simulink model "Boat_Simulation_Current_demo"  (R2015a)
settings: Solver=ode3  StartTime=0.0  StopTime=50  FixedStep=dt  RelTol=1e-3
values from neighbouring files (symbols this model uses):
  airfoil_lookup = [flip(aifoil_negative_side,1);airfoil_lookup]    [boatVars.m]
  allow_disable = 1    [boatVars.m]
  ay = depth_boat*l_boat    (= 0.0096)    [boatVars.m]
  cte_disable_thresh = 100    [boatVars.m]
  d_com_aero = 0.1    [boatVars.m]
  d_motors = w_boat-0.02    (= 0.06)    [boatVars.m]
  dt = 0.1    [Analytic_Field.m]    (also in Baseline_on_Sim.m = 0.0666666666667; TrackExample.m = 0.0666666666667; TrackExample_revised.m = 0.0666666666667; boatVars.m = 0.01)
  dtor = pi/180    (= 0.0174532925199)    [boatVars.m]
  Izz_a = rho_water*((l_boat/2)^2-(w_boat/2)^2)^2*depth_boat    (= 0.0013824)    [boatVars.m]
  Izz_boat = 1    [boatVars.m]
  k_drag_rot = 0.4    [boatVars.m]
  m_boat = 0.120    (= 0.12)    [boatVars.m]
  ma_x = pi*rho_water*(w_boat/2)^2*(depth_boat)    (= 0.301592894745)    [boatVars.m]
  ma_y = pi*rho_water*(l_boat/2)^2*(depth_boat)    (= 1.20637157898)    [boatVars.m]
  rho_water = 1000    [boatVars.m]
  rot_disable_thresh = 0.0    (= 0)    [boatVars.m]
  rtod = 180/pi    (= 57.2957795131)    [boatVars.m]
  s = size(im)    [ParticleFinder.m]    (also in efficientPath.m = [50 50]; efficientPathFunc.m = [26 12]; efficientPath_newGyre.m = [s/200.*[lambda_field b_field]]; efficientPath_trials.m = [yy/2 yy/2])
  waypoints = zeros(num_waypoints,2)    [efficientPath.m]    (also in efficientPathFunc.m; efficientPath_newGyre.m)
  xd = part_pos_2(ii-1,1)    [Baseline_on_Sim.m]    (also in TrackExample.m; TrackExample_revised.m; boatVars.m = 1.5)
  xs = linspace(0,lambda_field,nx)    [boatVars.m]    (also in efficientPath_trials.m = 0:xStep:2*yy; grid_define.m = xmin:step:xmax)
  yd = part_pos_2(ii-1,2)    [Baseline_on_Sim.m]    (also in TrackExample.m; TrackExample_revised.m; boatVars.m = 0.5)
  ys = linspace(0,b_field,ny)    [boatVars.m]    (also in efficientPath_trials.m = 0:yStep:yy; grid_define.m = ymin:step:ymax)
undefined symbols (not defined in the file or in its folder): m, thrust_disable_thresh
undefined symbols (not defined in the file): alpha0_boat, b_motor, J_motor, kphi_motor, L_motor, R_motor, theta0_boat, theta_dot0_boat, v0_boat_mag, x0_boat
libraries: simulink x7, aerolib3dof2 x3, aerolibutil x2, dspmathops x2, aerolibconvert2 x2, aerolib3dofsys x1
settings Model: Creator=Jack  LastModifiedBy=Jack

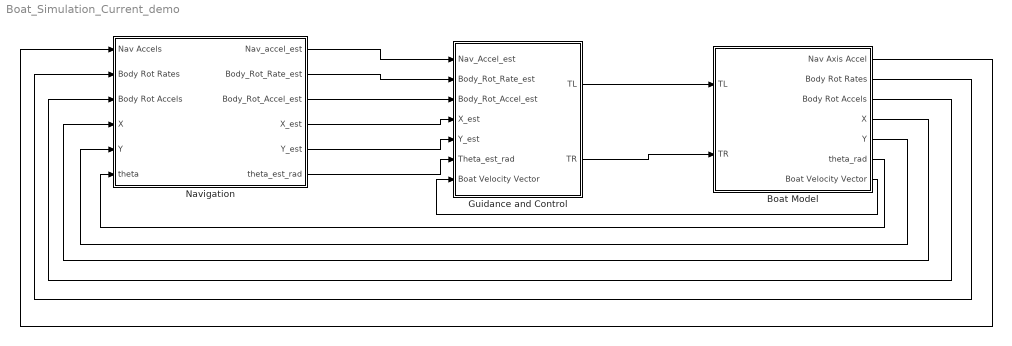
== system Boat_Simulation_Current_demo ==
  Boat Model : Subsystem
  Guidance and Control : Subsystem
  Navigation : Subsystem
  wires:
  Boat Model/1(Nav Axis Accel) -> Navigation/1(Nav Accels)
  Boat Model/2(Body Rot Rates) -> Navigation/2(Body Rot Rates)
  Boat Model/3(Body Rot Accels) -> Navigation/3(Body Rot Accels)
  Guidance and Control/1(TL) -> Boat Model/1(TL)
  Guidance and Control/2(TR) -> Boat Model/2(TR)
  Boat Model/4(X) -> Navigation/4(X)
  Boat Model/5(Y) -> Navigation/5(Y)
  Navigation/4(X_est) -> Guidance and Control/4(X_est)
  Navigation/5(Y_est) -> Guidance and Control/5(Y_est)
  Navigation/6(theta_est_rad) -> Guidance and Control/6(Theta_est_rad)
  Boat Model/6(theta_rad) -> Navigation/6(theta)
  Navigation/1(Nav_accel_est) -> Guidance and Control/1(Nav_Accel_est)
  Navigation/2(Body_Rot_Rate_est) -> Guidance and Control/2(Body_Rot_Rate_est)
  Navigation/3(Body_Rot_Accel_est) -> Guidance and Control/3(Body_Rot_Accel_est)
  Boat Model/7(Boat Velocity Vector) -> Guidance and Control/7(Boat Velocity Vector)

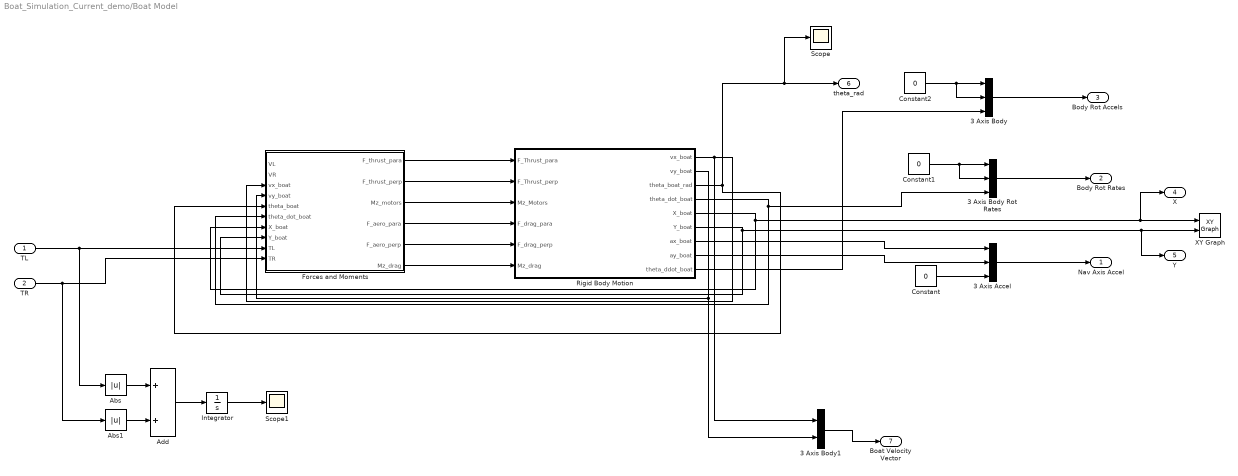
== system Boat_Simulation_Current_demo/Boat Model ==
  TL : Inport
  TR : Inport  Port=2
  3 Axis Accel : Concatenate  NumInputs=3
  3 Axis Body : Concatenate  NumInputs=3
  3 Axis Body Rot Rates : Concatenate  NumInputs=3
  3 Axis Body1 : Concatenate
  Abs : Abs
  Abs1 : Abs
  Add : Sum
  Constant : Constant  Value=0
  Constant1 : Constant  Value=0
  Constant2 : Constant  Value=0
  Forces and Moments : Subsystem
  Integrator : Integrator
  Rigid Body Motion : Subsystem
  Scope : Scope
      settings: TimeRange=10  YMin=2.71473  YMax=3.00049  SaveName=ScopeData5
  Scope1 : Scope
      settings: SaveName=ScopeData9
  XY Graph : simulink/Sinks/XY Graph  xmin=0  xmax=2  ymin=0  ymax=1  st=dt
  Nav Axis Accel : Outport
  Body Rot Rates : Outport  Port=2
  Body Rot Accels : Outport  Port=3
  X : Outport  Port=4
  Y : Outport  Port=5
  theta_rad : Outport  Port=6
  Boat Velocity Vector : Outport  Port=7
  wires:
  Forces and Moments/3(Mz_motors) -> Rigid Body Motion/3(Mz_Motors)
  Forces and Moments/2(F_thrust_perp) -> Rigid Body Motion/2(F_Thrust_perp)
  Forces and Moments/1(F_thrust_para) -> Rigid Body Motion/1(F_Thrust_para)
  Forces and Moments/4(F_aero_para) -> Rigid Body Motion/4(F_drag_para)
  Forces and Moments/5(F_aero_perp) -> Rigid Body Motion/5(F_drag_perp)
  Forces and Moments/6(Mz_drag) -> Rigid Body Motion/6(Mz_drag)
  Rigid Body Motion/1(vx_boat) -> 3 Axis Body1/1, Forces and Moments/3(vx_boat)
  Rigid Body Motion/2(vy_boat) -> 3 Axis Body1/2, Forces and Moments/4(vy_boat)
  Rigid Body Motion/3(theta_boat_rad) -> Forces and Moments/5(theta_boat), Scope/1, theta_rad/1
  Rigid Body Motion/4(theta_dot_boat) -> 3 Axis Body Rot Rates/3, Forces and Moments/6(theta_dot_boat)
  Rigid Body Motion/5(X_boat) -> Forces and Moments/7(X_boat), X/1, XY Graph/1
  Rigid Body Motion/6(Y_boat) -> Forces and Moments/8(Y_boat), Y/1, XY Graph/2
  Rigid Body Motion/7(ax_boat) -> 3 Axis Accel/1
  3 Axis Accel/1 -> Nav Axis Accel/1
  Rigid Body Motion/8(ay_boat) -> 3 Axis Accel/2
  Constant/1 -> 3 Axis Accel/3
  3 Axis Body Rot Rates/1 -> Body Rot Rates/1
  Constant1/1 -> 3 Axis Body Rot Rates/2, 3 Axis Body Rot Rates/1
  3 Axis Body/1 -> Body Rot Accels/1
  Constant2/1 -> 3 Axis Body/2, 3 Axis Body/1
  Rigid Body Motion/9(theta_ddot_boat) -> 3 Axis Body/3
  3 Axis Body1/1 -> Boat Velocity Vector/1
  TL/1 -> Abs/1, Forces and Moments/9(TL)
  TR/1 -> Abs1/1, Forces and Moments/10(TR)
  Abs/1 -> Add/1
  Abs1/1 -> Add/2
  Add/1 -> Integrator/1
  Integrator/1 -> Scope1/1

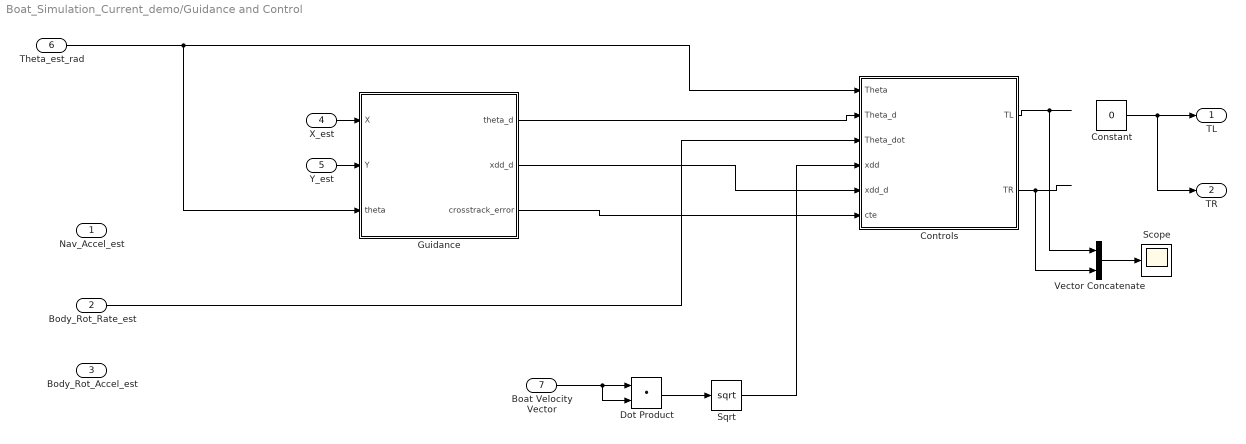
== system Boat_Simulation_Current_demo/Guidance and Control ==
  Nav_Accel_est : Inport
  Body_Rot_Rate_est : Inport  Port=2
  Body_Rot_Accel_est : Inport  Port=3
  X_est : Inport  Port=4
  Y_est : Inport  Port=5
  Theta_est_rad : Inport  Port=6
  Boat Velocity Vector : Inport  Port=7
  Constant : Constant  Value=0
  Controls : Subsystem
  Dot Product : DotProduct  InputSameDT=on  OutDataTypeStr=Inherit: Inherit via internal rule
  Guidance : Subsystem
  Scope : Scope
      settings: SaveName=ScopeData4
  Sqrt : Sqrt  SaturateOnIntegerOverflow=on
  Vector Concatenate : Concatenate
  TL : Outport
  TR : Outport  Port=2
  wires:
  Controls/1(TL) -> Vector Concatenate/1
  Controls/2(TR) -> Vector Concatenate/2
  X_est/1 -> Guidance/1(X)
  Y_est/1 -> Guidance/2(Y)
  Guidance/1(theta_d) -> Controls/2(Theta_d)
  Guidance/2(xdd_d) -> Controls/5(xdd_d)
  Theta_est_rad/1 -> Controls/1(Theta), Guidance/3(theta)
  Body_Rot_Rate_est/1 -> Controls/3(Theta_dot)
  Sqrt/1 -> Controls/4(xdd)
  Boat Velocity Vector/1 -> Dot Product/2, Dot Product/1
  Dot Product/1 -> Sqrt/1
  Vector Concatenate/1 -> Scope/1
  Guidance/3(crosstrack_error) -> Controls/6(cte)
  Constant/1 -> TR/1, TL/1

== system Boat_Simulation_Current_demo/Navigation ==
  Nav Accels : Inport
  Body Rot Rates : Inport  Port=2
  Body Rot Accels : Inport  Port=3
  X : Inport  Port=4
  Y : Inport  Port=5
  theta : Inport  Port=6
  Nav_accel_est : Outport
  Body_Rot_Rate_est : Outport  Port=2
  Body_Rot_Accel_est : Outport  Port=3
  X_est : Outport  Port=4
  Y_est : Outport  Port=5
  theta_est_rad : Outport  Port=6
  wires:
  X/1 -> X_est/1
  Y/1 -> Y_est/1
  theta/1 -> theta_est_rad/1
  Body Rot Accels/1 -> Body_Rot_Accel_est/1
  Body Rot Rates/1 -> Body_Rot_Rate_est/1
  Nav Accels/1 -> Nav_accel_est/1

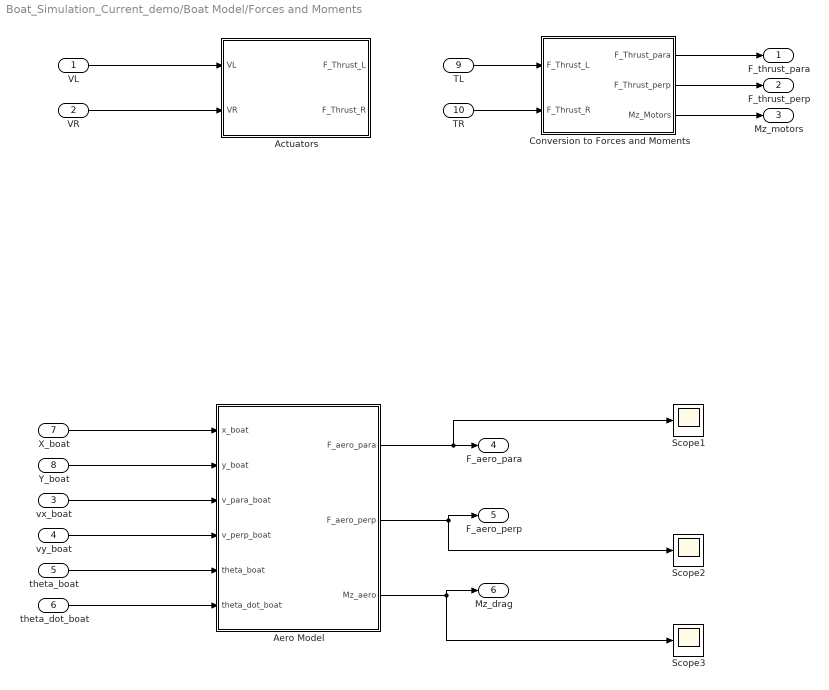
== system Boat_Simulation_Current_demo/Boat Model/Forces and Moments ==
  VL : Inport
  VR : Inport  Port=2
  vx_boat : Inport  Port=3
  vy_boat : Inport  Port=4
  theta_boat : Inport  Port=5
  theta_dot_boat : Inport  Port=6
  X_boat : Inport  Port=7
  Y_boat : Inport  Port=8
  TL : Inport  Port=9
  TR : Inport  Port=10
  Actuators : Subsystem
  Aero Model : Subsystem
  Conversion to Forces and Moments : Subsystem
  Scope1 : Scope
      settings: SaveName=ScopeData6
  Scope2 : Scope
      settings: TimeRange=10  SaveName=ScopeData8
  Scope3 : Scope
      settings: TimeRange=10  SaveName=ScopeData19
  F_thrust_para : Outport
  F_thrust_perp : Outport  Port=2
  Mz_motors : Outport  Port=3
  F_aero_para : Outport  Port=4
  F_aero_perp : Outport  Port=5
  Mz_drag : Outport  Port=6
  wires:
  VR/1 -> Actuators/2(VR)
  VL/1 -> Actuators/1(VL)
  Aero Model/3(Mz_aero) -> Scope3/1, Mz_drag/1
  Conversion to Forces and Moments/1(F_Thrust_para) -> F_thrust_para/1
  Conversion to Forces and Moments/2(F_Thrust_perp) -> F_thrust_perp/1
  Conversion to Forces and Moments/3(Mz_Motors) -> Mz_motors/1
  theta_dot_boat/1 -> Aero Model/6(theta_dot_boat)
  TL/1 -> Conversion to Forces and Moments/1(F_Thrust_L)
  TR/1 -> Conversion to Forces and Moments/2(F_Thrust_R)
  Aero Model/1(F_aero_para) -> Scope1/1, F_aero_para/1
  Aero Model/2(F_aero_perp) -> Scope2/1, F_aero_perp/1
  theta_boat/1 -> Aero Model/5(theta_boat)
  vy_boat/1 -> Aero Model/4(v_perp_boat)
  vx_boat/1 -> Aero Model/3(v_para_boat)
  Y_boat/1 -> Aero Model/2(y_boat)
  X_boat/1 -> Aero Model/1(x_boat)

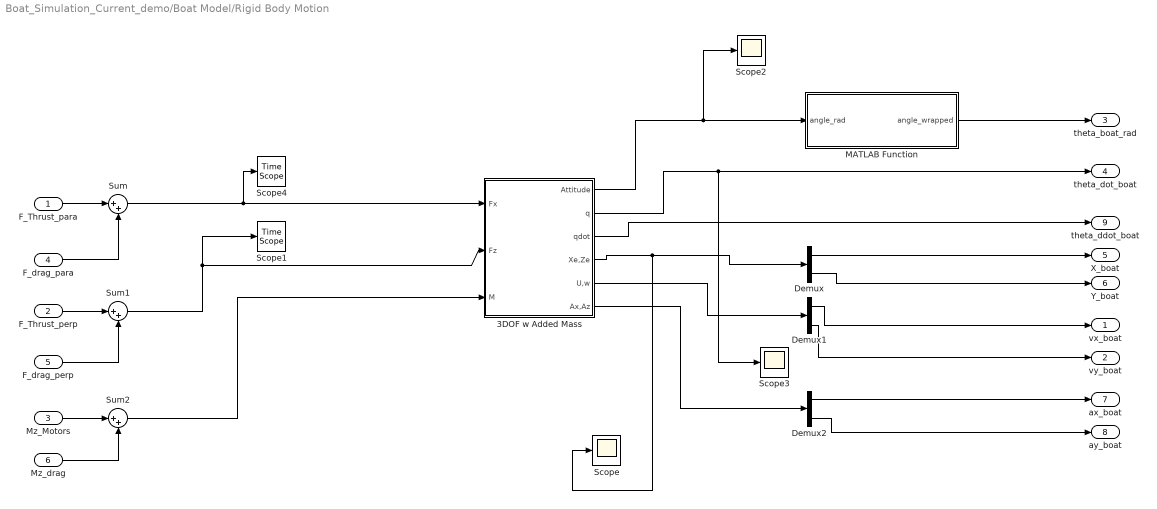
== system Boat_Simulation_Current_demo/Boat Model/Rigid Body Motion ==
  F_Thrust_para : Inport
  F_Thrust_perp : Inport  Port=2
  Mz_Motors : Inport  Port=3
  F_drag_para : Inport  Port=4
  F_drag_perp : Inport  Port=5
  Mz_drag : Inport  Port=6
  3DOF w Added Mass : Subsystem  mask(3DOF EoM){units=Metric (MKS), mtype=Fixed, v_ini=v0_boat_mag, theta_ini=theta0_boat, alpha_ini=alpha0_boat, q_ini=theta_dot0_boat, pos_ini=x0_boat, mass=m_boat, mass_e=0.5, mass_f=3.0, Iyy=Izz_boat, Iyy_e=0.5, Iyy_f=3.0, g_in=Internal, g=0, vre_flag=off}
      mask prompts: mtype "Mass type:"; v_ini "Initial velocity:"; theta_ini "Initial body attitude:"; alpha_ini "Initial incidence:"; q_ini "Initial body rotation rate:"; pos_ini "Initial position (x z):"; mass "Initial mass:"; mass_e "Empty mass:"; mass_f "Full mass:"; Iyy "Inertia:"; Iyy_e "Empty inertia:"; Iyy_f "Full inertia:"; g_in "Gravity source:"; g "Acceleration due to gravity:"; vre_flag "Include mass flow relative velocity"
      mask help: Integrate the three-degrees-of-freedom equations of motion to determine body position, velocity, attitude, and related values.
      mask init:
      | U0 = v_ini*cos(alpha_ini);
      | w0 = v_ini*sin(alpha_ini);
      | ports=aeroicon('aeroblk3dofbody','icon');
      mask Help: eval('asbhelp(''threedof_body_axes'')');
      mask TypeOptions units: Metric (MKS) | English (Velocity in ft/s) | English (Velocity in kts)
      mask TypeOptions mtype: Fixed | Simple Variable | Custom Variable
      mask Callback mtype: aeroicon('aeroblk3dofbody');
      mask TypeOptions g_in: Internal | External
      mask Callback g_in: aeroicon('aeroblk3dofbody');
      mask Display:
      | port_label(ports(1).type,ports(1).port,ports(1).txt,'texmode','on');
      | port_label(ports(2).type,ports(2).port,ports(2).txt,'texmode','on');
      | port_label(ports(3).type,ports(3).port,ports(3).txt,'texmode','on');
      | port_label(ports(4).type,ports(4).port,ports(4).txt,'texmode','on');
      | port_label(ports(5).type,ports(5).port,ports(5).txt,'texmode','on');
      | port_label(ports(6).type,ports(6).port,ports(6).txt,'texmode','on');
      | port_label(ports(7).type,ports(7).port,ports(7).txt,'texmode','on');
      | port_label(ports(8).type,ports(8).port,ports(8).txt,'texmode','on');
      | port_label(ports(9).type,ports(9).port,ports(9).txt,'texmode','on');
      | port_label(ports(10).type,ports(10).port,ports(10).txt,'texmode','on');
      | port_label(ports(11).type,ports(11).port,ports(11).txt,'texmode','on');
      | port_label(ports(12).type,ports(12).port,ports(12).txt,'texmode','on');
      | port_label(ports(13).type,ports(13).port,ports(13).txt,'texmode','on');
      | port_label(ports(14).type,ports(14).port,ports(14).txt,'texmode','on');
      | port_label(ports(15).type,ports(15).port,ports(15).txt,'texmode','on');
      | port_label(ports(16).type,ports(16).port,ports(16).txt,'texmode','on');
      | [x y xp yp highstr lowstr maxy miny]=aeroimage('threedofbody',gcbh);
      | plot(x,y);
      | patch(xp, yp);
      | text(0.5,maxy+0.08,highstr{:},'horizontalAlignment','center')
      | text(0.5,miny-0.05,lowstr{:},'horizontalAlignment','center')
  Demux : Demux  Outputs=2
  Demux1 : Demux  Outputs=2
  Demux2 : Demux  Outputs=2
  MATLAB Function : MATLAB Function  TreatAsAtomicUnit=on
  Scope : Scope
      settings: YMin=0  YMax=2
  Scope1 : TimeScope
  Scope2 : Scope
      settings: SaveName=ScopeData31
  Scope3 : Scope
      settings: SaveName=ScopeData32
  Scope4 : TimeScope
  Sum : Sum  Inputs=|++
  Sum1 : Sum  Inputs=|++
  Sum2 : Sum  Inputs=|++
  vx_boat : Outport
  vy_boat : Outport  Port=2
  theta_boat_rad : Outport  Port=3
  theta_dot_boat : Outport  Port=4
  X_boat : Outport  Port=5
  Y_boat : Outport  Port=6
  ax_boat : Outport  Port=7
  ay_boat : Outport  Port=8
  theta_ddot_boat : Outport  Port=9
  wires:
  F_drag_para/1 -> Sum/2
  Mz_Motors/1 -> Sum2/1
  Mz_drag/1 -> Sum2/2
  Demux/1 -> X_boat/1
  Demux/2 -> Y_boat/1
  Demux1/1 -> vx_boat/1
  Demux1/2 -> vy_boat/1
  Demux2/1 -> ax_boat/1
  Demux2/2 -> ay_boat/1
  MATLAB Function/1(angle_wrapped) -> theta_boat_rad/1
  3DOF w Added Mass/2("q ") -> Scope3/1, theta_dot_boat/1
  3DOF w Added Mass/3(qdot) -> theta_ddot_boat/1
  3DOF w Added Mass/1(Attitude) -> Scope2/1, MATLAB Function/1(angle_rad)
  3DOF w Added Mass/4(Xe,Ze) -> Scope/1, Demux/1
  3DOF w Added Mass/5("U,w  ") -> Demux1/1
  3DOF w Added Mass/6(Ax,Az) -> Demux2/1
  F_drag_perp/1 -> Sum1/2
  F_Thrust_para/1 -> Sum/1
  F_Thrust_perp/1 -> Sum1/1
  Sum1/1 -> Scope1/1, 3DOF w Added Mass/2(Fz)
  Sum/1 -> 3DOF w Added Mass/1(Fx), Scope4/1
  Sum2/1 -> 3DOF w Added Mass/3(M)

== system Boat_Simulation_Current_demo/Guidance and Control/Controls ==
  Theta : Inport
  Theta_d : Inport  Port=2
  Theta_dot : Inport  Port=3
  xdd : Inport  Port=4
  xdd_d : Inport  Port=5
  cte : Inport  Port=6
  Axial Control Loops : Subsystem
  Demux : Demux  Outputs=3
  Prop Allocation : Subsystem
  Rotation Control Loops : Subsystem
  TL : Outport
  TR : Outport  Port=2
  wires:
  Theta/1 -> Rotation Control Loops/1(Theta)
  Theta_d/1 -> Rotation Control Loops/2(Theta_d)
  Rotation Control Loops/1(Theta_err) -> Prop Allocation/1(theta_err)
  Prop Allocation/1(TL) -> TL/1
  Prop Allocation/2(TR) -> TR/1
  Axial Control Loops/1(xdd_err) -> Prop Allocation/2(xdd_err)
  xdd/1 -> Axial Control Loops/1(xdd)
  xdd_d/1 -> Axial Control Loops/2(xdd_d)
  Theta_dot/1 -> Demux/1
  Demux/3 -> Rotation Control Loops/3(Theta_dot_est)
  cte/1 -> Prop Allocation/3(cte)

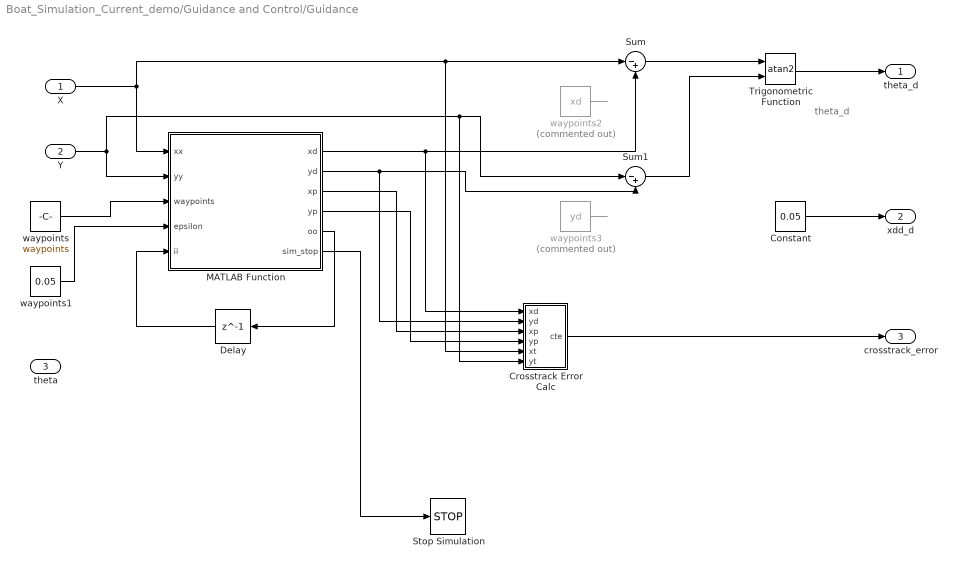
== system Boat_Simulation_Current_demo/Guidance and Control/Guidance ==
  note: theta_d
  X : Inport
  Y : Inport  Port=2
  theta : Inport  Port=3
  Constant : Constant  Value=0.05
  "Crosstrack Error Calc " : Subsystem
  Delay : Delay  DelayLength=1  InitialCondition=2
  MATLAB Function : MATLAB Function  TreatAsAtomicUnit=on
  Stop Simulation : Stop
  Sum : Sum  Inputs=|-+
  Sum1 : Sum  Inputs=|-+
  Trigonometric Function : Trigonometry  Operator=atan2
  waypoints : Constant  Value=waypoints
  waypoints1 : Constant  Value=0.05
  waypoints2 : Constant  Commented=on  Value=xd
  waypoints3 : Constant  Commented=on  Value=yd
  theta_d : Outport
  xdd_d : Outport  Port=2
  crosstrack_error : Outport  Port=3
  wires:
  X/1 -> MATLAB Function/1(xx), "Crosstrack Error Calc "/5(xt), Sum/1
  MATLAB Function/1(xd) -> Sum/2, "Crosstrack Error Calc "/1(xd)
  Sum/1 -> Trigonometric Function/1
  Sum1/1 -> Trigonometric Function/2
  Trigonometric Function/1 -> theta_d/1
  Constant/1 -> xdd_d/1
  waypoints/1 -> MATLAB Function/3(waypoints)
  waypoints1/1 -> MATLAB Function/4(epsilon)
  MATLAB Function/5(oo) -> Delay/1
  Delay/1 -> MATLAB Function/5(ii)
  waypoints2/1 -> ?
  waypoints3/1 -> ?
  MATLAB Function/6(sim_stop) -> Stop Simulation/1
  MATLAB Function/2(yd) -> Sum1/2, "Crosstrack Error Calc "/2(yd)
  MATLAB Function/3(xp) -> "Crosstrack Error Calc "/3(xp)
  MATLAB Function/4(yp) -> "Crosstrack Error Calc "/4(yp)
  "Crosstrack Error Calc "/1(cte) -> crosstrack_error/1
  Y/1 -> MATLAB Function/2(yy), "Crosstrack Error Calc "/6(yt), Sum1/1

== system Boat_Simulation_Current_demo/Boat Model/Forces and Moments/Actuators ==
  note: Left Motor
  note: Right Motor
  VL : Inport
  VR : Inport  Port=2
  DC motor : Subsystem  mask(DC Motor){L=L_motor, Kphi=kphi_motor, J=J_motor, b=b_motor, R=R_motor}
      mask help:
      | Takes the DC voltage as input, and outputs angular velocity (w) and current (i)
      | L => windings inductance		Kphi => emf constant
      | J => loads moment of inertial		b => viscous friction
      | R => windings resistance
      mask Display:
      | port_label('input', 1, 'V')
      | port_label('output', 2, 'i')
      | port_label('output', 1, 'w')
      | disp('DC Motor')
  DC motor1 : Subsystem  mask(DC Motor){L=L_motor, Kphi=kphi_motor, J=J_motor, b=b_motor, R=R_motor}
      mask help:
      | Takes the DC voltage as input, and outputs angular velocity (w) and current (i)
      | L => windings inductance		Kphi => emf constant
      | J => loads moment of inertial		b => viscous friction
      | R => windings resistance
      mask Display:
      | port_label('input', 1, 'V')
      | port_label('output', 2, 'i')
      | port_label('output', 1, 'w')
      | disp('DC Motor')
  Prop Angular Velocity to Thrust : Lookup_n-D  NumberOfTableDimensions=1  BreakpointsForDimension1=[-5:5]  Table=tanh([-5:5])  InternalRulePriority=Speed  RndMeth=Simplest  InputSameDT=on
  Prop Angular Velocity to Thrust1 : Lookup_n-D  NumberOfTableDimensions=1  BreakpointsForDimension1=[-5:5]  Table=tanh([-5:5])  InternalRulePriority=Speed  RndMeth=Simplest  InputSameDT=on
  F_Thrust_L : Outport
  F_Thrust_R : Outport  Port=2
  wires:
  DC motor/1(w) -> Prop Angular Velocity to Thrust/1
  DC motor1/1(w) -> Prop Angular Velocity to Thrust1/1
  VL/1 -> DC motor/1(V)
  VR/1 -> DC motor1/1(V)
  Prop Angular Velocity to Thrust/1 -> F_Thrust_L/1
  Prop Angular Velocity to Thrust1/1 -> F_Thrust_R/1

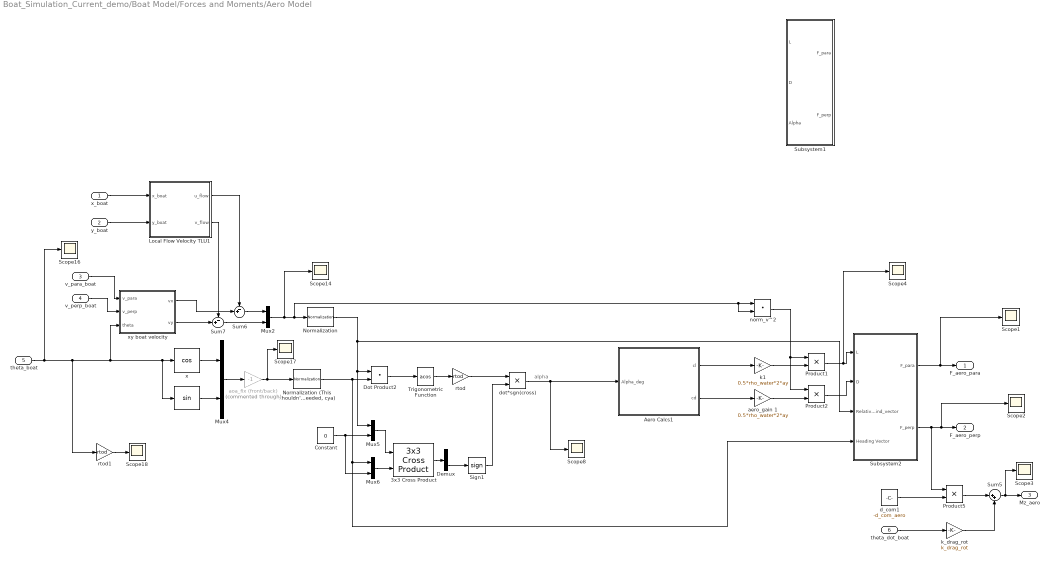
== system Boat_Simulation_Current_demo/Boat Model/Forces and Moments/Aero Model ==
  note: alpha
  x_boat : Inport
  y_boat : Inport  Port=2
  v_para_boat : Inport  Port=3
  v_perp_boat : Inport  Port=4
  theta_boat : Inport  Port=5
  theta_dot_boat : Inport  Port=6
  " " : Trigonometry
  3x3 Cross Product : aerolibutil/3x3 Cross Product
  Aero Calcs1 : Subsystem
  Constant : Constant  Value=0
  Demux : Demux  Outputs=3
  Dot Product2 : DotProduct  InputSameDT=on  OutDataTypeStr=Inherit: Inherit via internal rule
  Local Flow Velocity TLU1 : Subsystem
  Mux{2,4..6} (4 alike) : Mux  Inputs=2
  Normalization : dspmathops/Normalization  NormType=2-norm  Bias=1e-10  NormOver=Each column  ColComp=off  Dimension=1  outputDataTypeStr=Inherit: Same as product output  outputLastDataTypeStr=Inherit: Same as product output  outputMin=[]  outputMax=[]  accumDataTypeStr=Inherit: Same as product output  accumLastDataTypeStr=Inherit: Same as product output  roundingMode=Floor  overflowMode=off
  "Normalization (This shouldn't be needed, cya)" : dspmathops/Normalization  NormType=2-norm  Bias=1e-10  NormOver=Each column  ColComp=off  Dimension=1  outputDataTypeStr=Inherit: Same as product output  outputLastDataTypeStr=Inherit: Same as product output  outputMin=[]  outputMax=[]  accumDataTypeStr=Inherit: Same as product output  accumLastDataTypeStr=Inherit: Same as product output  roundingMode=Floor  overflowMode=off
  Product1 : Product
  Product2 : Product
  Product5 : Product
  Scope{1..4,8,14,16..18} (9 alike) : Scope
      Scope1 settings: YMin=-0.000475  YMax=-0.000225  SaveName=ScopeData7
      Scope14 settings: ShowLegends=on  SaveName=ScopeData24
      Scope16 settings: SaveName=ScopeData28
      Scope17 settings: ShowLegends=on  SaveName=ScopeData29
      Scope18 settings: YMin=45  YMax=45  SaveName=ScopeData30
      Scope2 settings: YMin=-1  YMax=1  SaveName=ScopeData10
      Scope3 settings: YMin=-1  YMax=1  SaveName=ScopeData11
      Scope4 settings: ShowLegends=on  YMin=-0.005  YMax=0.075  SaveName=ScopeData16
      Scope8 settings: YMin=-141.75  YMax=-128.25  SaveName=ScopeData26
  Sign1 : Signum
  Subsystem1 : Subsystem
  Subsystem2 : Subsystem
  Sum5 : Sum  Inputs=|++
  Sum6 : Sum  Inputs=-+|
  Sum7 : Sum  Inputs=-+|
  Trigonometric Function : Trigonometry  Operator=acos
  aero_gain 1 : Gain  Gain=0.5*rho_water*2*ay
  aoa_fix (front/back) : Gain  Commented=through  Gain=-1
  d_com1 : Constant  Value=-d_com_aero
  dot*sgn(cross) : Product
  k1 : Gain  Gain=0.5*rho_water*2*ay
  k_drag_rot : Gain  Gain=k_drag_rot
  norm_v^2 : DotProduct  InputSameDT=on  OutDataTypeStr=Inherit: Inherit via internal rule
  rtod : Gain  Gain=rtod
  rtod1 : Gain  Gain=rtod
  x : Trigonometry  Operator=cos
  "xy boat velocity " : Subsystem
  F_aero_para : Outport
  F_aero_perp : Outport  Port=2
  Mz_aero : Outport  Port=3
  wires:
  x_boat/1 -> Local Flow Velocity TLU1/1(x_boat)
  y_boat/1 -> Local Flow Velocity TLU1/2(y_boat)
  Local Flow Velocity TLU1/1(u_flow) -> Sum6/1
  Local Flow Velocity TLU1/2(v_flow) -> Sum7/1
  theta_dot_boat/1 -> k_drag_rot/1
  k_drag_rot/1 -> Sum5/2
  Subsystem2/2(F_perp) -> Product5/1, Scope2/1, F_aero_perp/1
  d_com1/1 -> Product5/2
  Product5/1 -> Sum5/1
  Sum5/1 -> Scope3/1, Mz_aero/1
  theta_boat/1 -> Scope16/1, rtod1/1, "xy boat velocity "/3("theta "), " "/1, x/1
  x/1 -> Mux4/1
  " "/1 -> Mux4/2
  Mux2/1 -> Scope14/1, norm_v^2/2, norm_v^2/1, Normalization/1
  Mux4/1 -> aoa_fix (front/back)/1
  "Normalization (This shouldn't be needed, cya)"/1 -> Subsystem2/4(Heading Vector), Mux6/1, Dot Product2/2
  Dot Product2/1 -> Trigonometric Function/1
  Trigonometric Function/1 -> rtod/1
  rtod/1 -> dot*sgn(cross)/1
  Normalization/1 -> Mux5/1, Dot Product2/1, Subsystem2/3(Relative_wind_vector)
  v_para_boat/1 -> "xy boat velocity "/1(v_para)
  v_perp_boat/1 -> "xy boat velocity "/2(v_perp)
  "xy boat velocity "/1(vx) -> Sum6/2
  "xy boat velocity "/2(vy) -> Sum7/2
  Sum6/1 -> Mux2/1
  Sum7/1 -> Mux2/2
  rtod1/1 -> Scope18/1
  Constant/1 -> Mux6/2, Mux5/2
  Mux5/1 -> 3x3 Cross Product/1
  Mux6/1 -> 3x3 Cross Product/2
  Sign1/1 -> dot*sgn(cross)/2
  dot*sgn(cross)/1 -> Scope8/1, Aero Calcs1/1(Alpha_deg)
  3x3 Cross Product/1 -> Demux/1
  Demux/3 -> Sign1/1
  Aero Calcs1/1(cl) -> k1/1
  k1/1 -> Product1/2
  aero_gain 1/1 -> Product2/2
  norm_v^2/1 -> Product2/1, Product1/1
  Aero Calcs1/2(cd) -> aero_gain 1/1
  Product1/1 -> Scope4/1, Subsystem2/1(L)
  Product2/1 -> Subsystem2/2(D)
  aoa_fix (front/back)/1 -> Scope17/1, "Normalization (This shouldn't be needed, cya)"/1
  Subsystem2/1(F_para) -> Scope1/1, F_aero_para/1

== system Boat_Simulation_Current_demo/Boat Model/Forces and Moments/Conversion to Forces and Moments ==
  F_Thrust_L : Inport
  F_Thrust_R : Inport  Port=2
  Constant : Constant  Value=0
  Divide : Product  Inputs=*/
  Sum : Sum  Inputs=|++
  Sum1 : Sum  Inputs=+-|
  d_motors/2 : Constant  Value=d_motors/2
  F_Thrust_para : Outport
  F_Thrust_perp : Outport  Port=2
  Mz_Motors : Outport  Port=3
  wires:
  F_Thrust_L/1 -> Sum1/1, Sum/1
  F_Thrust_R/1 -> Sum1/2, Sum/2
  Sum/1 -> F_Thrust_para/1
  Constant/1 -> F_Thrust_perp/1
  Sum1/1 -> Divide/1
  d_motors/2/1 -> Divide/2
  Divide/1 -> Mz_Motors/1

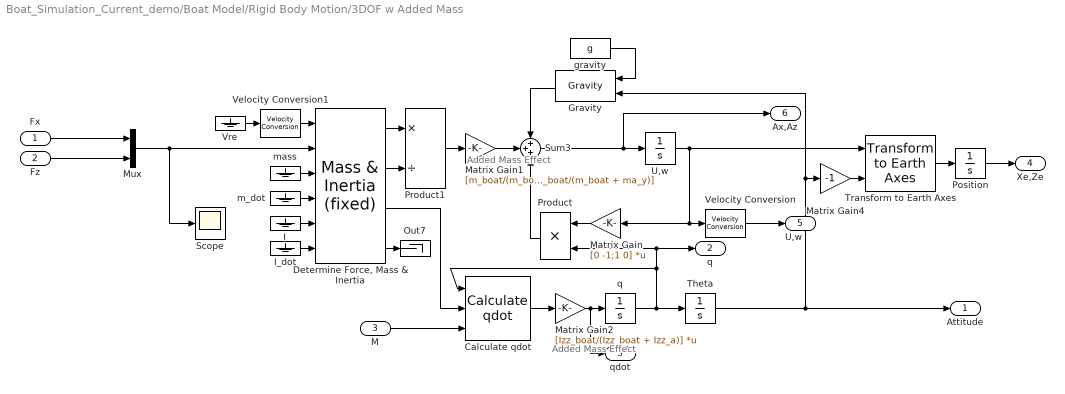
== system Boat_Simulation_Current_demo/Boat Model/Rigid Body Motion/3DOF w Added Mass ==
  note: Added
      | Mass
      | Effect
  note: Added
      | Mass
      | Effect
  Fx : Inport
  Fz : Inport  Port=2
  M : Inport  Port=3
  Calculate qdot : aerolib3dof2/3DOF (Body Axes)/Calculate qdot
  "Determine Force, Mass & Inertia" : aerolib3dofsys/Mass & Inertia (fixed)  SystemSampleTime=-1
  Gravity : aerolib3dof2/3DOF (Body Axes)/Gravity
  I : Ground
  I_dot : Ground
  Matrix Gain : Gain  Gain=[0 -1;1 0]  Multiplication=Matrix(K*u)  SaturateOnIntegerOverflow=on  OutDataTypeStr=Inherit: Same as input  ParamDataTypeStr=Inherit: Same as input
  Matrix Gain1 : Gain  Gain=[m_boat/(m_boat + ma_x); m_boat/(m_boat + ma_y)]  SaturateOnIntegerOverflow=on  OutDataTypeStr=Inherit: Same as input  ParamDataTypeStr=Inherit: Same as input
  Matrix Gain2 : Gain  Gain=[Izz_boat/(Izz_boat + Izz_a)]  Multiplication=Matrix(K*u)  SaturateOnIntegerOverflow=on  OutDataTypeStr=Inherit: Same as input  ParamDataTypeStr=Inherit: Same as input
  Matrix Gain4 : Gain  Gain=-1  SaturateOnIntegerOverflow=on  OutDataTypeStr=Inherit: Same as input  ParamDataTypeStr=Inherit: Same as input
  Mux : Mux  Inputs=2
  Out7 : Terminator
  Position : Integrator  InitialCondition=pos_ini
  Product : Product  SaturateOnIntegerOverflow=on  InputSameDT=on  OutDataTypeStr=Inherit: Same as first input
  Product1 : Product  Inputs=*/  SaturateOnIntegerOverflow=on  OutDataTypeStr=Inherit: Same as first input
  Scope : Scope
      settings: ShowLegends=on  SaveName=ScopeData33
  Sum3 : Sum  Inputs=+++  SaturateOnIntegerOverflow=on
  Theta : Integrator  InitialCondition=theta_ini
  Transform to Earth Axes : aerolib3dof2/3DOF (Body Axes)/Transform  to Earth Axes
  U,w : Integrator  InitialCondition=convvel([U0 w0],'m/s','m/s')
  Velocity Conversion : aerolibconvert2/Velocity Conversion  IU=m/s  OU=m/s
  Velocity Conversion1 : aerolibconvert2/Velocity Conversion  IU=m/s  OU=m/s
  Vre : Ground
  gravity : Constant  Value=g  OutDataTypeStr=Inherit: Inherit via back propagation
  m_dot : Ground
  mass : Ground
  q : Integrator  InitialCondition=q_ini
  Attitude : Outport  InitialOutput=0
  "q " : Outport  Port=2  InitialOutput=0
  qdot : Outport  Port=3  InitialOutput=0
  Xe,Ze : Outport  Port=4  InitialOutput=0
  "U,w  " : Outport  Port=5  InitialOutput=0
  Ax,Az : Outport  Port=6  InitialOutput=0
  wires:
  U,w/1 -> Velocity Conversion/1, Matrix Gain/1, Transform to Earth Axes/1
  Velocity Conversion/1 -> "U,w  "/1
  Velocity Conversion1/1 -> "Determine Force, Mass & Inertia"/1
  Vre/1 -> Velocity Conversion1/1
  "Determine Force, Mass & Inertia"/4 -> Out7/1
  q/1 -> Calculate qdot/1, Product/2, "q "/1, Theta/1
  I_dot/1 -> "Determine Force, Mass & Inertia"/6
  mass/1 -> "Determine Force, Mass & Inertia"/3
  "Determine Force, Mass & Inertia"/1 -> Product1/1
  "Determine Force, Mass & Inertia"/2 -> Product1/2
  gravity/1 -> Gravity/1
  m_dot/1 -> "Determine Force, Mass & Inertia"/4
  I/1 -> "Determine Force, Mass & Inertia"/5
  Position/1 -> Xe,Ze/1
  "Determine Force, Mass & Inertia"/3 -> Calculate qdot/2
  Gravity/1 -> Sum3/1
  Transform to Earth Axes/1 -> Position/1
  Fx/1 -> Mux/1
  Mux/1 -> Scope/1, "Determine Force, Mass & Inertia"/2
  Matrix Gain/1 -> Product/1
  Product/1 -> Sum3/3
  Product1/1 -> Matrix Gain1/1
  Matrix Gain1/1 -> Sum3/2
  Calculate qdot/1 -> Matrix Gain2/1
  Matrix Gain2/1 -> qdot/1, q/1
  Sum3/1 -> Ax,Az/1, U,w/1
  Fz/1 -> Mux/2
  Theta/1 -> Attitude/1, Matrix Gain4/1, Gravity/2
  Matrix Gain4/1 -> Transform to Earth Axes/2
  M/1 -> Calculate qdot/3

== system Boat_Simulation_Current_demo/Guidance and Control/Controls/Axial Control Loops ==
  xdd : Inport
  xdd_d : Inport  Port=2
  PID Controller : simulink/Continuous/PID Controller  Controller=PID  TimeDomain=Continuous-time  SampleTime=-1  IntegratorMethod=Forward Euler  FilterMethod=Forward Euler  Form=Parallel  UseFilter=on  ControllerParametersSource=internal  P=2  I=0  D=0  N=1  InitialConditionSource=internal  InitialConditionForIntegrator=0  InitialConditionForFilter=0  ExternalReset=none  LimitOutput=off  UpperSaturationLimit=inf  LowerSaturationLimit=-inf  LinearizeAsGain=on  AntiWindupMode=none  Kb=1  TrackingMode=off  Kt=1  PParamMin=[]  PParamMax=[]  IParamMin=[]  IParamMax=[]  DParamMin=[]  DParamMax=[]  NParamMin=[]  NParamMax=[]  KbParamMin=[]  KbParamMax=[]  KtParamMin=[]  KtParamMax=[]  POutMin=[]  POutMax=[]  IOutMin=[]  IOutMax=[]  DOutMin=[]  DOutMax=[]  NOutMin=[]  NOutMax=[]  KbOutMin=[]  KbOutMax=[]  KtOutMin=[]  KtOutMax=[]  IntegratorOutMin=[]  IntegratorOutMax=[]  FilterOutMin=[]  FilterOutMax=[]  SumOutMin=[]  SumOutMax=[]  SumI1OutMin=[]  SumI1OutMax=[]  SumI2OutMin=[]  SumI2OutMax=[]  SumI3OutMin=[]  SumI3OutMax=[]  SumDOutMin=[]  SumDOutMax=[]  SaturationOutMin=[]  SaturationOutMax=[]  IntegratorContinuousStateAttributes=''  IntegratorStateMustResolveToSignalObject=off  IntegratorRTWStateStorageClass=Auto  FilterContinuousStateAttributes=''  FilterStateMustResolveToSignalObject=off  FilterRTWStateStorageClass=Auto  DifferentiatorICPrevScaledInput=0  DifferentiatorOutMin=[]  DifferentiatorOutMax=[]
  Scope : Scope
      settings: SaveName=ScopeData3
  Sum : Sum  Inputs=|++
  xdd_err : Outport
  wires:
  xdd/1 -> Sum/1
  xdd_d/1 -> Sum/2
  PID Controller/1 -> Scope/1, xdd_err/1
  Sum/1 -> PID Controller/1

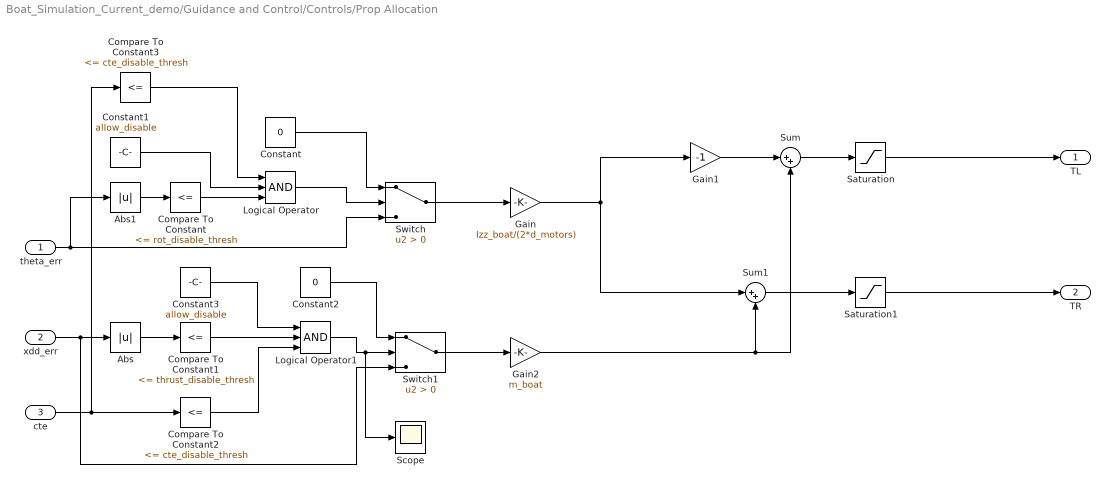
== system Boat_Simulation_Current_demo/Guidance and Control/Controls/Prop Allocation ==
  theta_err : Inport
  xdd_err : Inport  Port=2
  cte : Inport  Port=3
  Abs : Abs
  Abs1 : Abs
  Compare To Constant : simulink/Logic and Bit Operations/Compare To Constant  relop=<=  const=rot_disable_thresh  OutDataTypeStr=boolean
  Compare To Constant1 : simulink/Logic and Bit Operations/Compare To Constant  relop=<=  const=thrust_disable_thresh  OutDataTypeStr=boolean
  Compare To Constant2 : simulink/Logic and Bit Operations/Compare To Constant  relop=<=  const=cte_disable_thresh  OutDataTypeStr=boolean
  Compare To Constant3 : simulink/Logic and Bit Operations/Compare To Constant  relop=<=  const=cte_disable_thresh  OutDataTypeStr=boolean
  Constant : Constant  Value=0
  Constant1 : Constant  Value=allow_disable
  Constant2 : Constant  Value=0
  Constant3 : Constant  Value=allow_disable
  Gain : Gain  Gain=Izz_boat/(2*d_motors)
  Gain1 : Gain  Gain=-1
  Gain2 : Gain  Gain=m_boat
  Logical Operator : Logic  Inputs=3  AllPortsSameDT=off  OutDataTypeStr=boolean
  Logical Operator1 : Logic  Inputs=3  AllPortsSameDT=off  OutDataTypeStr=boolean
  Saturation : Saturate  UpperLimit=0.2  LowerLimit=-0.2
  Saturation1 : Saturate  UpperLimit=0.3  LowerLimit=-0.3
  Scope : Scope
      settings: SaveName=ScopeData12
  Sum : Sum  Inputs=|++
  Sum1 : Sum  Inputs=|++
  Switch : Switch  Criteria=u2 > Threshold
  Switch1 : Switch  Criteria=u2 > Threshold
  TL : Outport
  TR : Outport  Port=2
  wires:
  theta_err/1 -> Switch/3, Abs1/1
  Gain/1 -> Sum1/1, Gain1/1
  Gain1/1 -> Sum/1
  Gain2/1 -> Sum1/2, Sum/2
  Sum/1 -> Saturation/1
  Sum1/1 -> Saturation1/1
  Saturation/1 -> TL/1
  Saturation1/1 -> TR/1
  Switch/1 -> Gain/1
  Logical Operator/1 -> Switch/2
  Constant/1 -> Switch/1
  Constant1/1 -> Logical Operator/2
  Compare To Constant/1 -> Logical Operator/3
  xdd_err/1 -> Switch1/3, Abs/1
  Switch1/1 -> Gain2/1
  Logical Operator1/1 -> Scope/1, Switch1/2
  Constant2/1 -> Switch1/1
  Constant3/1 -> Logical Operator1/1
  Compare To Constant1/1 -> Logical Operator1/2
  Abs/1 -> Compare To Constant1/1
  Abs1/1 -> Compare To Constant/1
  cte/1 -> Compare To Constant3/1, Compare To Constant2/1
  Compare To Constant2/1 -> Logical Operator1/3
  Compare To Constant3/1 -> Logical Operator/1

== system Boat_Simulation_Current_demo/Guidance and Control/Controls/Rotation Control Loops ==
  Theta : Inport
  Theta_d : Inport  Port=2
  Theta_dot_est : Inport  Port=3
  Constant : Constant  Value=-pi/2
  MATLAB Function : MATLAB Function  TreatAsAtomicUnit=on
  Mux : Mux  Inputs=3
  PID Controller : simulink/Continuous/PID Controller  Controller=PID  TimeDomain=Continuous-time  SampleTime=-1  IntegratorMethod=Forward Euler  FilterMethod=Forward Euler  Form=Parallel  UseFilter=on  ControllerParametersSource=internal  P=1  I=0  D=0  N=0  InitialConditionSource=internal  InitialConditionForIntegrator=0  InitialConditionForFilter=0  ExternalReset=none  LimitOutput=off  UpperSaturationLimit=inf  LowerSaturationLimit=-inf  LinearizeAsGain=on  AntiWindupMode=none  Kb=1  TrackingMode=off  Kt=1  PParamMin=[]  PParamMax=[]  IParamMin=[]  IParamMax=[]  DParamMin=[]  DParamMax=[]  NParamMin=[]  NParamMax=[]  KbParamMin=[]  KbParamMax=[]  KtParamMin=[]  KtParamMax=[]  POutMin=[]  POutMax=[]  IOutMin=[]  IOutMax=[]  DOutMin=[]  DOutMax=[]  NOutMin=[]  NOutMax=[]  KbOutMin=[]  KbOutMax=[]  KtOutMin=[]  KtOutMax=[]  IntegratorOutMin=[]  IntegratorOutMax=[]  FilterOutMin=[]  FilterOutMax=[]  SumOutMin=[]  SumOutMax=[]  SumI1OutMin=[]  SumI1OutMax=[]  SumI2OutMin=[]  SumI2OutMax=[]  SumI3OutMin=[]  SumI3OutMax=[]  SumDOutMin=[]  SumDOutMax=[]  SaturationOutMin=[]  SaturationOutMax=[]  IntegratorContinuousStateAttributes=''  IntegratorStateMustResolveToSignalObject=off  IntegratorRTWStateStorageClass=Auto  FilterContinuousStateAttributes=''  FilterStateMustResolveToSignalObject=off  FilterRTWStateStorageClass=Auto  DifferentiatorICPrevScaledInput=0  DifferentiatorOutMin=[]  DifferentiatorOutMax=[]
  Scope2 : Scope
      settings: ShowLegends=on  MaxDataPoints=100000
  Sum1 : Sum  Inputs=++|
  Sum2 : Sum  Inputs=|++
  dt : Gain  Gain=dt
  k_drag_rot : Gain  Gain=k_drag_rot
  Theta_err : Outport
  wires:
  PID Controller/1 -> Theta_err/1
  MATLAB Function/1(err) -> Mux/1, Sum1/2
  Theta_d/1 -> Sum2/1
  Theta/1 -> MATLAB Function/1(theta), Mux/2
  Theta_dot_est/1 -> k_drag_rot/1
  k_drag_rot/1 -> dt/1
  dt/1 -> Sum1/1
  Sum1/1 -> PID Controller/1
  Constant/1 -> Sum2/2
  Sum2/1 -> Mux/3, MATLAB Function/2(theta_d)
  Mux/1 -> Scope2/1

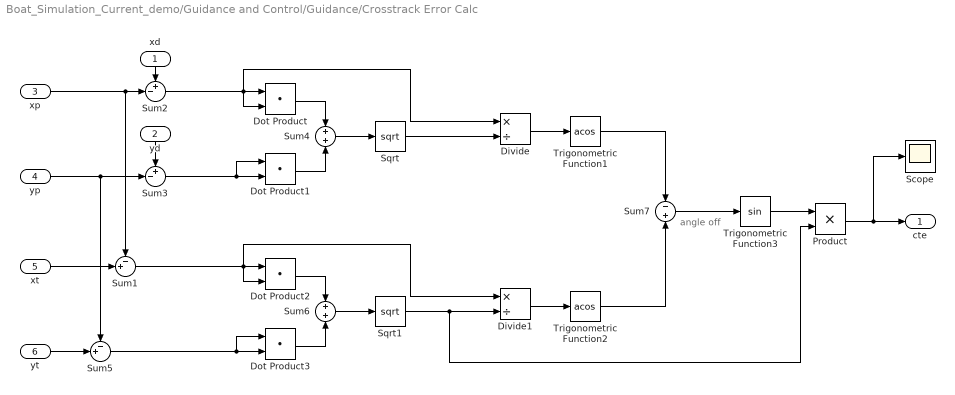
== system Boat_Simulation_Current_demo/Guidance and Control/Guidance/Crosstrack Error Calc  ==
  note: angle off
  xd : Inport
  yd : Inport  Port=2
  xp : Inport  Port=3
  yp : Inport  Port=4
  xt : Inport  Port=5
  yt : Inport  Port=6
  Divide : Product  Inputs=*/
  Divide1 : Product  Inputs=*/
  Dot Product{,1..3} (4 alike) : DotProduct  InputSameDT=on  OutDataTypeStr=Inherit: Inherit via internal rule
  Product : Product
  Scope : Scope
      settings: SaveName=ScopeData2
  Sqrt : Sqrt  SaturateOnIntegerOverflow=on
  Sqrt1 : Sqrt  SaturateOnIntegerOverflow=on
  Sum1 : Sum  Inputs=-+|
  Sum2 : Sum  Inputs=+-|
  Sum3 : Sum  Inputs=+-|
  Sum4 : Sum  Inputs=+|+
  Sum5 : Sum  Inputs=-+|
  Sum6 : Sum  Inputs=+|+
  Sum7 : Sum  Inputs=-|+
  Trigonometric Function1 : Trigonometry  Operator=acos
  Trigonometric Function2 : Trigonometry  Operator=acos
  Trigonometric Function3 : Trigonometry
  cte : Outport
  wires:
  Divide/1 -> Trigonometric Function1/1
  Trigonometric Function1/1 -> Sum7/1
  Sum4/1 -> Sqrt/1
  Dot Product1/1 -> Sum4/2
  Dot Product/1 -> Sum4/1
  Sqrt/1 -> Divide/2
  Sum3/1 -> Dot Product1/1, Dot Product1/2
  xd/1 -> Sum2/1
  yd/1 -> Sum3/1
  Sum2/1 -> Divide/1, Dot Product/2, Dot Product/1
  xt/1 -> Sum1/2
  yt/1 -> Sum5/2
  Divide1/1 -> Trigonometric Function2/1
  Trigonometric Function2/1 -> Sum7/2
  Sum6/1 -> Sqrt1/1
  Dot Product3/1 -> Sum6/2
  Dot Product2/1 -> Sum6/1
  Sqrt1/1 -> Product/2, Divide1/2
  Sum5/1 -> Dot Product3/1, Dot Product3/2
  xp/1 -> Sum2/2, Sum1/1
  yp/1 -> Sum3/2, Sum5/1
  Sum1/1 -> Divide1/1, Dot Product2/2, Dot Product2/1
  Sum7/1 -> Trigonometric Function3/1
  Trigonometric Function3/1 -> Product/1
  Product/1 -> Scope/1, cte/1

== system Boat_Simulation_Current_demo/Boat Model/Forces and Moments/Actuators/DC motor ==
  note: i
  note: w
  V : Inport
  1/ J : Gain  Gain=1/J
  1/ L : Gain  Gain=1/L
  Integrator1 : Integrator
  Integrator2 : Integrator
  Kphi : Gain  Gain=Kphi
  "Kphi " : Gain  Gain=Kphi
  R : Gain  Gain=R
  Sum : Sum  Inputs=|+--
  Sum1 : Sum  Inputs=|+-
  b : Gain  Gain=b
  w : Outport
  i : Outport  Port=2
  wires:
  V/1 -> Sum/1
  Sum/1 -> 1/ L/1
  1/ L/1 -> Integrator2/1
  Integrator2/1 -> Kphi/1, R/1, i/1
  Kphi/1 -> Sum1/1
  Sum1/1 -> 1/ J/1
  1/ J/1 -> Integrator1/1
  Integrator1/1 -> "Kphi "/1, b/1, w/1
  b/1 -> Sum1/2
  "Kphi "/1 -> Sum/3
  R/1 -> Sum/2

== system Boat_Simulation_Current_demo/Boat Model/Forces and Moments/Actuators/DC motor1 ==
  note: i
  note: w
  V : Inport
  1/ J : Gain  Gain=1/J
  1/ L : Gain  Gain=1/L
  Integrator1 : Integrator
  Integrator2 : Integrator
  Kphi : Gain  Gain=Kphi
  "Kphi " : Gain  Gain=Kphi
  R : Gain  Gain=R
  Sum : Sum  Inputs=|+--
  Sum1 : Sum  Inputs=|+-
  b : Gain  Gain=b
  w : Outport
  i : Outport  Port=2
  wires:
  V/1 -> Sum/1
  Sum/1 -> 1/ L/1
  1/ L/1 -> Integrator2/1
  Integrator2/1 -> Kphi/1, R/1, i/1
  Kphi/1 -> Sum1/1
  Sum1/1 -> 1/ J/1
  1/ J/1 -> Integrator1/1
  Integrator1/1 -> "Kphi "/1, b/1, w/1
  b/1 -> Sum1/2
  "Kphi "/1 -> Sum/3
  R/1 -> Sum/2

== system Boat_Simulation_Current_demo/Boat Model/Forces and Moments/Aero Model/Aero Calcs1 ==
  Alpha_deg : Inport
  cd lookup : Lookup_n-D  NumberOfTableDimensions=1  BreakpointsForDimension1=airfoil_lookup(:,1)  BeginIndexSearchUsingPreviousIndexResult=on  Table=airfoil_lookup(:,3)  ExtrapMethod=Clip  UseLastTableValue=on  InternalRulePriority=Speed  RndMeth=Simplest  InputSameDT=on
  cl lookup : Lookup_n-D  NumberOfTableDimensions=1  BreakpointsForDimension1=airfoil_lookup(:,1)  BeginIndexSearchUsingPreviousIndexResult=on  Table=airfoil_lookup(:,2)  ExtrapMethod=Clip  UseLastTableValue=on  InternalRulePriority=Speed  RndMeth=Simplest  InputSameDT=on
  cl : Outport
  cd : Outport  Port=2
  wires:
  cl lookup/1 -> cl/1
  cd lookup/1 -> cd/1
  Alpha_deg/1 -> cd lookup/1, cl lookup/1

== system Boat_Simulation_Current_demo/Boat Model/Forces and Moments/Aero Model/Local Flow Velocity TLU1 ==
  x_boat : Inport
  y_boat : Inport  Port=2
  U_field : Lookup_n-D  BreakpointsForDimension1=xs  BreakpointsForDimension2=ys  BeginIndexSearchUsingPreviousIndexResult=on  Table=U_field'  ExtrapMethod=Clip  UseLastTableValue=on  InternalRulePriority=Speed  RndMeth=Simplest  InputSameDT=on
  V_field : Lookup_n-D  BreakpointsForDimension1=xs  BreakpointsForDimension2=ys  BeginIndexSearchUsingPreviousIndexResult=on  Table=V_field_load'  ExtrapMethod=Clip  UseLastTableValue=on  InternalRulePriority=Speed  RndMeth=Simplest  InputSameDT=on
  u_flow : Outport
  v_flow : Outport  Port=2
  wires:
  U_field/1 -> u_flow/1
  V_field/1 -> v_flow/1
  x_boat/1 -> U_field/1, V_field/1
  y_boat/1 -> V_field/2, U_field/2

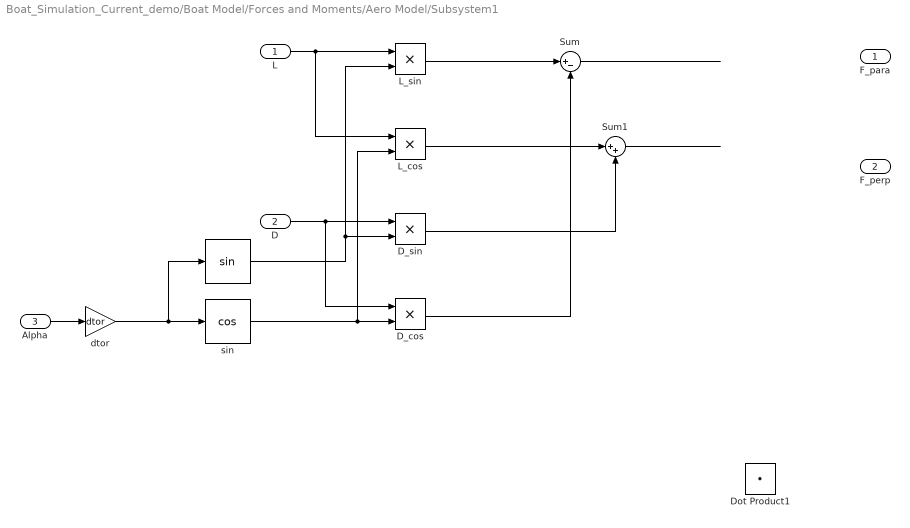
== system Boat_Simulation_Current_demo/Boat Model/Forces and Moments/Aero Model/Subsystem1 ==
  L : Inport
  D : Inport  Port=2
  Alpha : Inport  Port=3
  " " : Trigonometry
  D_cos : Product  Inputs=**
  D_sin : Product  Inputs=**
  Dot Product1 : DotProduct  InputSameDT=on  OutDataTypeStr=Inherit: Inherit via internal rule
  L_cos : Product  Inputs=**
  L_sin : Product  Inputs=**
  Sum : Sum  Inputs=|+-
  Sum1 : Sum  Inputs=|++
  dtor : Gain  Gain=dtor
  sin : Trigonometry  Operator=cos
  F_para : Outport
  F_perp : Outport  Port=2
  wires:
  " "/1 -> D_sin/2, L_sin/2
  sin/1 -> D_cos/2, L_cos/2
  L_cos/1 -> Sum1/1
  L_sin/1 -> Sum/1
  Alpha/1 -> dtor/1
  dtor/1 -> " "/1, sin/1
  L/1 -> L_cos/1, L_sin/1
  D_cos/1 -> Sum/2
  D_sin/1 -> Sum1/2
  D/1 -> D_cos/1, D_sin/1
  Sum/1 -> ?
  Sum1/1 -> ?

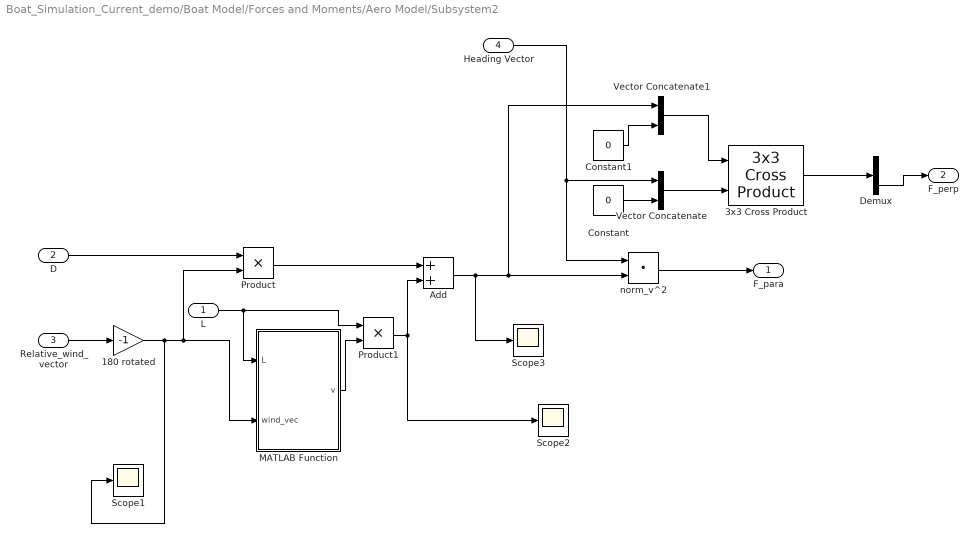
== system Boat_Simulation_Current_demo/Boat Model/Forces and Moments/Aero Model/Subsystem2 ==
  L : Inport
  D : Inport  Port=2
  Relative_wind_vector : Inport  Port=3
  Heading Vector : Inport  Port=4
  180 rotated : Gain  Gain=-1
  3x3 Cross Product : aerolibutil/3x3 Cross Product
  Add : Sum
  Constant : Constant  Value=0
  Constant1 : Constant  Value=0
  Demux : Demux  Outputs=3
  MATLAB Function : MATLAB Function  TreatAsAtomicUnit=on
  Product : Product
  Product1 : Product
  Scope1 : Scope
      settings: ShowLegends=on  YMin=-0.005  YMax=0.075  SaveName=ScopeData14
  Scope2 : Scope
      settings: ShowLegends=on  YMin=-1.5  YMax=1.5  SaveName=ScopeData15
  Scope3 : Scope
      settings: ShowLegends=on  YMin=-0.1  YMax=0.075
  Vector Concatenate : Concatenate
  Vector Concatenate1 : Concatenate
  norm_v^2 : DotProduct  InputSameDT=on  OutDataTypeStr=Inherit: Inherit via internal rule
  F_para : Outport
  F_perp : Outport  Port=2
  wires:
  L/1 -> MATLAB Function/1(L), Product1/1
  D/1 -> Product/1
  Relative_wind_vector/1 -> 180 rotated/1
  Product/1 -> Add/1
  Add/1 -> Scope3/1, Vector Concatenate1/1, norm_v^2/2
  Vector Concatenate/1 -> 3x3 Cross Product/2
  Heading Vector/1 -> Vector Concatenate/1, norm_v^2/1
  norm_v^2/1 -> F_para/1
  Constant/1 -> Vector Concatenate/2
  Constant1/1 -> Vector Concatenate1/2
  3x3 Cross Product/1 -> Demux/1
  Demux/3 -> F_perp/1
  MATLAB Function/1(v) -> Product1/2
  Product1/1 -> Add/2, Scope2/1
  Vector Concatenate1/1 -> 3x3 Cross Product/1
  180 rotated/1 -> Scope1/1, MATLAB Function/2(wind_vec), Product/2

== system Boat_Simulation_Current_demo/Boat Model/Forces and Moments/Aero Model/xy boat velocity  ==
  v_para : Inport
  v_perp : Inport  Port=2
  "theta " : Inport  Port=3
  Sum6 : Sum  Inputs=|+-
  Sum7 : Sum  Inputs=|++
  Trigonometric Function : Trigonometry
  Trigonometric Function1 : Trigonometry  Operator=cos
  para_cos : Product
  para_sin : Product
  perp_cos : Product
  perp_sin : Product
  vx : Outport
  vy : Outport  Port=2
  wires:
  Sum7/1 -> vy/1
  v_perp/1 -> perp_sin/1, perp_cos/1
  Sum6/1 -> vx/1
  v_para/1 -> para_cos/1, para_sin/1
  "theta "/1 -> Trigonometric Function1/1, Trigonometric Function/1
  Trigonometric Function1/1 -> perp_cos/2, para_cos/2
  Trigonometric Function/1 -> perp_sin/2, para_sin/2
  para_sin/1 -> Sum7/1
  perp_cos/1 -> Sum7/2
  perp_sin/1 -> Sum6/2
  para_cos/1 -> Sum6/1

== matlab function Boat_Simulation_Current_demo/Guidance and Control/Controls/Rotation Control Loops/MATLAB Function ==
  data: theta input; err output; theta_d input
function err = turnCorrection(theta,theta_d)
    if (theta>0 && theta_d<0 && abs(theta-theta_d)>pi)
        err = -(2*pi-abs(theta-theta_d));
    elseif (theta<0 && theta_d>0 && abs(theta-theta_d)>pi)
        err = (2*pi-abs(theta-theta_d));
    else
        err = theta-theta_d;
    end
end

== matlab function Boat_Simulation_Current_demo/Boat Model/Rigid Body Motion/MATLAB Function ==
  data: angle_rad input; angle_wrapped output
function angle_wrapped = wrap2pi(angle_rad)
    angle_wrapped = angle_rad - 2*pi*floor( (angle_rad+pi)/(2*pi) ); 
end

== matlab function Boat_Simulation_Current_demo/Guidance and Control/Guidance/MATLAB Function ==
  data: xx input; yy input; waypoints input; epsilon input; ii input; xd output; yd output; xp output; yp output; oo output; sim_stop output
function [xd,yd,xp,yp,oo,sim_stop] = choose_waypoint(xx,yy,waypoints,epsilon,ii)
    sim_stop = 0;
    dist_to_lp_waypoint = norm([waypoints(ii,1)-xx,waypoints(ii,2)-yy]);
    if dist_to_lp_waypoint < epsilon
        oo = floor(ii+1);
        if oo>length(waypoints(:,1))
            sim_stop = 1;
            oo = oo-1;
        end
    else
        oo = floor(ii);
    end
    xd = waypoints(oo,1);
    yd = waypoints(oo,2);
    xp = waypoints(oo-1,1);
    yp = waypoints(oo-1,2);
end

== matlab function Boat_Simulation_Current_demo/Boat Model/Forces and Moments/Aero Model/Subsystem2/MATLAB Function ==
  data: L input; wind_vec input; v output
function v = lift_dir(L,wind_vec)
%#codegen
v = zeros(2,1);
if (wind_vec(1) >0 && L>0) || (wind_vec(1) <0 && L<0)
    v = [0 -1;1 0]*wind_vec;
else
    v = [0 1;-1 0]*wind_vec;
end
